simulink model "test_newfft_fun2"  (Simulink 6.2)
settings: Solver=ode45  StartTime=0.0  StopTime=3200.0  RelTol=1e-3
libraries: xbsIndex_r3 x643, simulink x1
(part 1 of 10)
settings Model: LastModifiedBy=mdexter  foo=bar
settings DebuggingCC: SolverPrmCheckMsg=warning

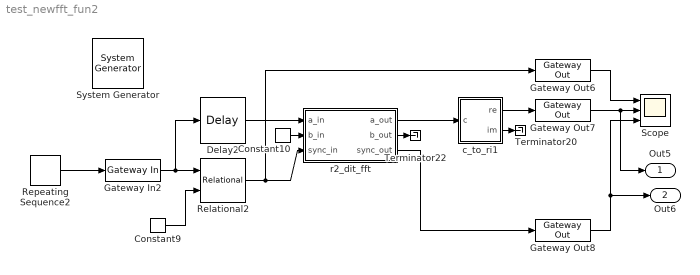
== system test_newfft_fun2 ==
  " System Generator" : xbsIndex_r3/ System Generator  Tag=genX  xilinxfamily=Virtex2  part=xc2v1000  speed=-4  package=bg575  synthesis_tool=XST  directory=./netlist  testbench=off  simulink_period=1  sysclk_period=100  incr_netlist=off  trim_vbits=Everywhere in SubSystem  dbl_ovrd=According to Block Masks  core_generation=According to Block Masks  run_coregen=off  deprecated_control=off  eval_field=0
      settings: AttributesFormatString=System\nGenerator
  Constant10 : xbsIndex_r3/Constant  const=0  equ=P=C  arith_type=Unsigned  n_bits=16  bin_pt=0  opselect=C  inp2=PCIN>>17  opr=+  inp1=P  carry=CIN  iostate=0  explicit_period=on  period=1  dbl_ovrd=off
  Constant9 : xbsIndex_r3/Constant  const=0  equ=P=C  arith_type=Unsigned  n_bits=16  bin_pt=0  opselect=C  inp2=PCIN>>17  opr=+  inp1=P  carry=CIN  iostate=0  explicit_period=on  period=1  dbl_ovrd=off
  Delay2 : xbsIndex_r3/Delay  latency=2  reg_retiming=off  explicit_period=off  period=1  en=off  accept_only_valid=off  init_zero=on  dbl_ovrd=off  show_param=off
      settings: xl_area=[0, 0, 0, 0, 0, 0, 0]
  Gateway In2 : xbsIndex_r3/Gateway In  arith_type=Unsigned  n_bits=16  bin_pt=0  quantization=Truncate  overflow=Wrap  period=1  timing_constraint=None  locs_specified=off  LOCs={}  needs_fixed_name=off  dbl_ovrd=off  show_param=off
      settings: xl_area=[0, 0, 0, 0, 0, 0, 0]
  Gateway Out6 : xbsIndex_r3/Gateway Out  output_type=Double  nbits=8  bin_pt=6  arith_type=Boolean  quantization=Truncate  overflow=Wrap  hdl_port=on  timing_constraint=None  locs_specified=off  LOCs={}  needs_fixed_name=off  show_param=off
      settings: xl_area=[0, 0, 0, 0, 0, 0, 0]
  Gateway Out7 : xbsIndex_r3/Gateway Out  output_type=Double  nbits=8  bin_pt=6  arith_type=Boolean  quantization=Truncate  overflow=Wrap  hdl_port=on  timing_constraint=None  locs_specified=off  LOCs={}  needs_fixed_name=off  show_param=off
      settings: xl_area=[0, 0, 0, 0, 0, 0, 0]
  Gateway Out8 : xbsIndex_r3/Gateway Out  output_type=Double  nbits=8  bin_pt=6  arith_type=Boolean  quantization=Truncate  overflow=Wrap  hdl_port=on  timing_constraint=None  locs_specified=off  LOCs={}  needs_fixed_name=off  show_param=off
      settings: xl_area=[0, 0, 0, 0, 0, 0, 0]
  Relational2 : xbsIndex_r3/Relational  mode=a!=b  latency=0  explicit_period=off  period=1  en=off  dbl_ovrd=off  show_param=off
      settings: xl_area=[0, 0, 0, 0, 0, 0, 0]
  Repeating Sequence2 : simulink/Sources/Repeating Sequence  rep_seq_t=[0:1024]  rep_seq_y=[1 zeros(1,1023) 1]*hex2dec('7f00')
  Scope : Scope  NumInputPorts=3
      settings: YMin=-5~-5~-5  YMax=5~5~5
  Terminator20 : Terminator
  Terminator22 : Terminator
  c_to_ri1 : Subsystem  mask(Complex to Real-Imag){n_bits=18, bin_pt=7}
      mask prompts: n_bits "Bit Width"; bin_pt "Binary Point"
      mask help: Outputs real and imaginary components of a complex input.
      mask init:
      | c_to_ri_init(gcb,n_bits,bin_pt);
      settings: AttributesFormatString=18_7 r/i
      mask Help:
      | <pre>
      | Description::
      | 
      | Outputs real and imaginary components of a complex input.
      | Useful for simplifying interconnects.
      | See also: Real-Imag to Complex (ri_to_c)
      | 
      | Mask Parameters::
      | 
      | Bit Width (n_bits): Specifies the width of the real/imaginary components.
      | Assumed equal for both components.
      | 
      | Binary Point (bin_pt): Specifies the binary point location in the real/imaginary components.
      | Assumed equal for both components.
      | </pre>
  r2_dit_fft : Subsystem  AncestorBlock=newfft_library/FFT/r2_dit_fft  mask(Biplex Radix-2 DIT FFT){n_stages=10, n_bits=8, bin_pt=7, shifts=[0], commutator_bram=0, twiddle_bram=0, n_bits_w=8, mult_latency=3, add_latency=1, commute_output=Yes (SLR16), output_order=Normal, show_sbo=on, munge_submasks=DumbDown}
      mask prompts: n_stages "Total Stages"; n_bits "Number of Bits In"; bin_pt "Binary Point In"; shifts "Shifting Schedule"; commutator_bram "Number of Stages Using BRAM for Biplex Commutators (i.e. delays)"; twiddle_bram "Number of Stages Using BRAM for Twiddle Coefficients"; n_bits_w "Twiddle Coefficient Bitwidth"; mult_latency "Multiplier Latency"; add_latency "Adder Latency"; commute_output "Commute Output"; output_order "Output Order"; show_sbo "Show Sub-Block Options"; munge_submasks "Sub-Block Masks"
      mask help: A biplex radix-2 decimation-in-time Fast Fourier Transform.
      mask init:
      | tic
      | r2_dit_fft_init(gcb, ...
      |   n_stages, ...
      |   n_bits, ...
      |   bin_pt, ...
      |   shifts, ...
      |   commutator_bram, ...
      |   twiddle_bram, ...
      |   n_bits_w, ...
      |   mult_latency, ...
      |   add_latency, ...
      |   commute_output, ...
      |   output_order, ...
      |   lower(get_param(gcb,'munge_submasks')) );
      | disp('r2_dit_fft initialization complete.');
      | toc
      settings: AttributesFormatString=|
      | 1024 points
      | 8_7 r/i in
      | 8_6 twiddles
      mask Help:
      | <pre>
      | Description::
      | 
      | A biplex radix-2 decimation-in-time Fast Fourier Transform.
      | 
      | The two inputs to the biplex FFT are independent complex signals (e.g. A and B).
      | 
      | Without an output commutator, the two outputs of the FFT are commuted such that the a_out
      | signal is really the "lower" half of A's transform followed by the "lower" half of B's
      | transform and b_out is really the "upper" half of A's transform followed by the "upper"
      | half of B's transform.
      | 
      | If it is desired to have the two halves of A's transform follow each other on the same path
      | and the two halves of B's transform follow each other on the same path, then be sure to
      | check the "Output Commutator" checkbox.  This will result in the "lower" half of A (or B)
      | followed by the "upper" half of A (or B).  Including the output commutator uses additional
      | resources.
      | 
      | If the "Normal" Ouput Order option is chosen, the output will be in normal order (though still in
      | commuted halves if no output commutator is used).  If the "Bit Reversed" Output Order" option is
      | selected, the output halves (either commuted or not) will each be in bit reversed order
      | (i.e. each half of each transform will be in bit reversed output order).   Normal output is easier
      | for humans to work with (especially for testing), but it uses additional resources.  Bit reversed
      | output is the implementation's inhernet output order so that option uses no additional resources.
      | 
      | The number of bits for each real and imaginary component grows by two through each stage.
      | If a stage's input bit width is 17 or less, three embedded multipliers will be used per complex multiply.
      | If a stage's input bit width is 18, four embedded multipliers will be used per complex multiply.
      | If a stage's input bit width exceeds 18, then substantially more embedded multipliers will be used
      | per complex multiply.  Enabling "shifting" in some (or all) stages can limit the bit growth
      | to prevent this.  See the Shifting Schedule parameter for more info.
      | 
      | Mask Parameters::
      | 
      | Total Stages (n_stages):  The number of total stages in the FFT.
      | The FFT will have 2^n_stages points.
      | 
      | Number of Bits In (n_bits): Specifies the width of the real/imaginary components of ports
      | a_in and b_in.  Assumed equal for both components.  The output bit width will be
      | n_bits+n_stages (assuming sum(shifts)==0).
      | 
      | Binary Point In (bin_pt): Specifies the binary point position of the real/imaginary
      | components of ports a_in and b_in.  Assumed equal for both components.
      | 
      | Shifting Schedule (shifts): A vector specifying how many bits to shift by at each stage.
      | Missing values are assumed to be zero; extra values are ignored.
      | 
      | Number of Stages Using BRAM for Biplex Commutators (commutator_bram): Number of stages
      | that will use BRAM for commutator memory.  Remaining stages will use SLR16 elements (slices).
      | 
      | Number of Stages Using BRAM for Twiddle Coefficients (twiddle_bram): Number of stages that
      | will use BRAM for twiddle coeeficient storage.  Remaining stages will use distributed memory
      | (slices).
      | 
      | Twiddle Coefficient Bitwidth (n_bits_w): Specifies the width of the real/imaginary
      | components of the twiddle coefficients.  Assumed equal for both components.
      | 
      | Multiplier Latency (mult_latency): Latency to use for the underlying real multipliers.
      | 
      | Adder Latency (add_latency): Latency to use for the underlying real adders.
      | 
      | Commute Output (commute_output): Popup options for an output commutator.  See decription
      | above for details on the output commutator.  Choices are:
      |     "No" - No output commutator
      |     "Yes (SLR16)" - Include output commutator using SLR16 elements
      |     "Yes (BRAM)" - Include output commutator using BRAM
      | 
      | Output Order (output_order): Popup options for selecting the output order.  See description
      | above for details on the output order.  Choices are:
      |     "Bit Reversed" - Output each half of each transform in bit reversed order.
      |     "Normal" - Output each half of each transform in normal order.
      | </pre>
      mask StyleString: edit,edit,edit,edit,edit,edit,edit,edit,edit,popup(No|Yes (SLR16)|Yes (BRAM)),popup(Bit Reversed|Normal),checkbox,popup(Keep|DumbDown|Unmask)
      mask CallbackString:
      | |||||||||||mvs=get_param(gcb,'MaskVisibilityString');
      | if strcmp(get_param(gcb,'show_sbo'),'on')
      |   onoff='on';
      | else
      |   onoff='off';
      | end
      | mvs=regexprep(mvs,'o[nf]*$',onoff);
      | set_param(gcb,'MaskVisibilityString',mvs);
      | |mvs=get_param(gcb,'MaskVisibilityString');
      | if strcmp(get_param(gcb,'show_sbo'),'on')
      |   onoff='on';
      | else
      |   onoff='off';
      | end
      | mvs=regexprep(mvs,'o[nf]*$',onoff);
      | set_param(gcb,'MaskVisibilityString',mvs);
  Out5 : Outport
  Out6 : Outport  Port=2
  wires:
  Relational2/1 -> Gateway Out6/1, r2_dit_fft/3(sync_in)
  Delay2/1 -> r2_dit_fft/1(a_in)
  Gateway In2/1 -> Relational2/1, Delay2/1
  Constant9/1 -> Relational2/2
  Gateway Out6/1 -> Scope/1
  Gateway Out7/1 -> Scope/2, Out5/1
  Gateway Out8/1 -> Out6/1, Scope/3
  Repeating Sequence2/1 -> Gateway In2/1
  r2_dit_fft/3(sync_out) -> Gateway Out8/1
  Constant10/1 -> r2_dit_fft/2(b_in)
  r2_dit_fft/1(a_out) -> c_to_ri1/1(c)
  c_to_ri1/1(re) -> Gateway Out7/1
  c_to_ri1/2(im) -> Terminator20/1
  r2_dit_fft/2(b_out) -> Terminator22/1

== system test_newfft_fun2/c_to_ri1 ==
  c : Inport  Port=1  LatchInput=off
  force_im : xbsIndex_r3/Reinterpret  force_arith_type=on  arith_type="Signed  (2's comp)"  force_bin_pt=on  bin_pt=7  force_valid=on
  force_re : xbsIndex_r3/Reinterpret  force_arith_type=on  arith_type="Signed  (2's comp)"  force_bin_pt=on  bin_pt=7  force_valid=on
  slice_im : xbsIndex_r3/Slice  mode=Lower Bit Location + Width  nbits=18  bit1=0  base1=MSB of Input  bit0=0  base0=LSB of Input  boolean_output=off  explicit_period=off  period=1  dbl_ovrd=off
  slice_re : xbsIndex_r3/Slice  mode=Upper Bit Location + Width  nbits=18  bit1=0  base1=MSB of Input  bit0=0  base0=LSB of Input  boolean_output=off  explicit_period=off  period=1  dbl_ovrd=off
  re : Outport
  im : Outport  Port=2
  wires:
  slice_re/1 -> force_re/1
  slice_im/1 -> force_im/1
  force_re/1 -> re/1
  force_im/1 -> im/1
  c/1 -> slice_re/1, slice_im/1
